simulink model "SSMM_sim_Torque_3DOF"  (R2020a)
settings: Solver=FixedStepAuto  StartTime=0.0  StopTime=120  FixedStep=0.001  MaxStep=1e-1  MinStep=1e-15  RelTol=.01  AbsTol=.01  EnableMultiTasking=on
InitFcn:
  | SSMM_sim_Torque_3DOF_Init
values from neighbouring files (symbols this model uses):
  CP_Num = CP_Base_Num + CP_Wheels_Num    [JACKAL_dynamic_model.m]
  D = D(:)    [ANFISFcn.m]    (also in JACKAL_dynamic_model.m = 1000)
  K = 1e6    (= 1000000)    [JACKAL_dynamic_model.m]
  model = floatbase(model)    [JACKAL_dynamic_model.m]
  Mu = .8    (= 0.8)    [JACKAL_dynamic_model.m]
  path = [      0         0 ... (first row only)    [JACKAL_dynamic_model.m]
  q_init = [0 0 0 0]'    [JACKAL_dynamic_model.m]
  qd_init = [0 0 0 0]'    [JACKAL_dynamic_model.m]
  R = .1    (= 0.1)    [JACKAL_dynamic_model.m]    (also in R.mat)
  speed = 1.5    [JACKAL_dynamic_model.m]
  width = basesize(2)    [JACKAL_dynamic_model.m]
  x_init = [1 0 0 0  0 0 zoff   0 0 0  2 0 0]'    [JACKAL_dynamic_model.m]
undefined symbols (not defined in the file or in its folder): DiscIntNeverNeededParam, Fpt, gcontact, gcPosVel
libraries: simulink x6, fuzblock x1
settings Model: Creator=Sergio  LastModifiedBy=sky32
settings SolverCC: MaxConsecutiveMinStep=5  AutoInsertRateTranBlk=on
settings DataIOCC: SaveFormat=Array  SignalLoggingSaveFormat=ModelDataLogs  ReturnWorkspaceOutputs=off
settings OptimizationCC: ExpressionDepthLimit=2147483647  LifeSpan=inf
settings DebuggingCC: UnderspecifiedInitializationDetection=Classic  MergeDetectMultiDrivingBlocksExec=none  SolverPrmCheckMsg=warning  MultiTaskDSMMsg=warning  MultiTaskCondExecSysMsg=none  StateNameClashWarn=warning  SFUnexpectedBacktrackingDiag=warning  SFNoUnconditionalDefaultTransitionDiag=warning  SFExecutionAtInitializationDiag=none  ArithmeticOperatorsInVariantConditions=warning
settings HardwareCC: ProdBitPerPointer=32  ProdBitPerSizeT=32  ProdBitPerPtrDiffT=32  ProdLargestAtomicFloat=None  ProdIntDivRoundTo=Undefined  ProdEndianess=Unspecified  ProdWordSize=32  ProdHWDeviceType=32-bit Generic
settings ModelReferenceCC: PropagateSignalLabelsOutOfModel=off
settings SFSimCC: SimUseLocalCustomCode=off  CustomCodeUndefinedFunction=UseInterfaceOnly
settings RTWCC: RTWUseLocalCustomCode=off
settings CodeAppCC: StateflowObjectComments=on
settings GRTTargetCC: TargetLangStandard=C89/C90 (ANSI)
settings ConfigComp: CovMetricSettings=dw  CovHtmlReporting=on  CovSaveCumulativeToWorkspaceVar=on  CovSaveSingleToWorkspaceVar=on  CovExternalEMLEnable=off

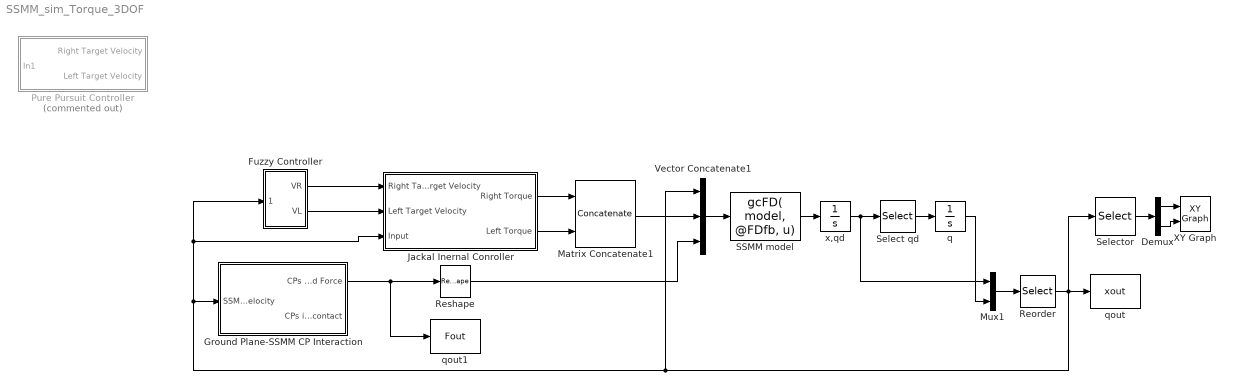
== system SSMM_sim_Torque_3DOF ==
  Demux : Demux  Outputs=2
  Fuzzy Controller : Subsystem
  Ground Plane-SSMM CP Interaction : Subsystem
  Jackal Inernal Conroller : Subsystem
  Matrix Concatenate1 : Concatenate  Mode=Multidimensional array
  Mux1 : Mux  Inputs=2
  Pure Pursuit Controller : Subsystem  Commented=on
  Reorder : Selector  InputPortWidth=21  IndexOptions=Index vector (dialog)  Indices=[1 2 3 4 5 6 7 8 9 10 11 12 13 18 19 20 21 14 15 16 17]  OutputSizes=1
  Reshape : Reshape  OutputDimensionality=Column vector (2-D)
  SSMM model : MATLABFcn  MATLABFcn=gcFD( model, @FDfb, u)  OutputDimensions=[17 1]  OutputSignalType=real  Output1D=off
  Select qd : Selector  InputPortWidth=17  IndexOptions=Index vector (dialog)  Indices=[14 15 16 17]  OutputSizes=1
  Selector : Selector  InputPortWidth=21  IndexOptions=Index vector (dialog)  Indices=[5 6]  OutputSizes=1
  Vector Concatenate1 : Concatenate  NumInputs=3
  XY Graph : simulink/Sinks/XY Graph  xmin=-10  xmax=20  ymin=-20  ymax=10  st=-1
  q : Integrator  InitialCondition=q_init
  qout : ToWorkspace  VariableName=xout  SampleTime=-1
  qout1 : ToWorkspace  VariableName=Fout  SampleTime=-1
  x,qd : Integrator  InitialCondition=[x_init;qd_init]
  wires:
  Vector Concatenate1/1 -> SSMM model/1
  SSMM model/1 -> x,qd/1
  Reshape/1 -> Vector Concatenate1/3
  x,qd/1 -> Select qd/1, Mux1/1
  Select qd/1 -> q/1
  Mux1/1 -> Reorder/1
  q/1 -> Mux1/2
  Ground Plane-SSMM CP Interaction/1(CPs Applied Force) -> qout1/1, Reshape/1
  Matrix Concatenate1/1 -> Vector Concatenate1/2
  Jackal Inernal Conroller/1(Right Torque) -> Matrix Concatenate1/1
  Jackal Inernal Conroller/2(Left Torque) -> Matrix Concatenate1/2
  Demux/2 -> XY Graph/2
  Selector/1 -> Demux/1
  Demux/1 -> XY Graph/1
  Reorder/1 -> Vector Concatenate1/1, Ground Plane-SSMM CP Interaction/1(SSMM Position and Velocity), Fuzzy Controller/1(theta,x,y), Jackal Inernal Conroller/3(Input), Selector/1, qout/1
  Fuzzy Controller/1(VR) -> Jackal Inernal Conroller/1(Right Target Velocity)
  Fuzzy Controller/2(VL) -> Jackal Inernal Conroller/2(Left Target Velocity)

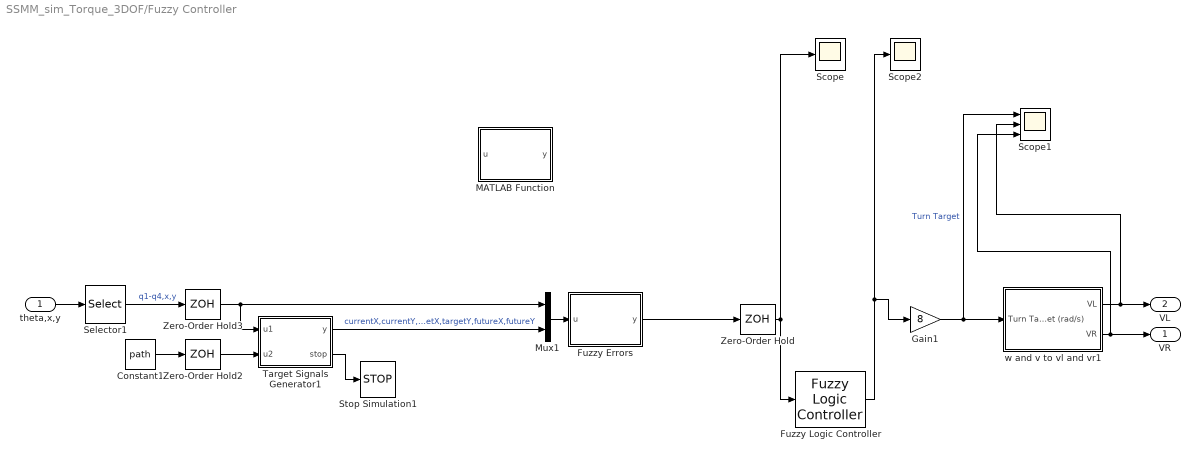
== system SSMM_sim_Torque_3DOF/Fuzzy Controller ==
  theta,x,y : Inport
  Constant1 : Constant  Value=path
  Fuzzy Errors : MATLAB Function  TreatAsAtomicUnit=on
  Fuzzy Logic Controller : fuzblock/Fuzzy Logic  Controller  FIS='fuzzycontrolthreeinputs6'  OutputSampleNumber=101  DataType=double  FuzzifiedInputs=off  RuleFiringStrengths=off  RuleOutputs=off  AggregatedOutputs=off  SimulateUsing=Interpreted execution  OutOfRangeInputValueMessage=warning  NoRuleFiredMessage=warning  EmptyOutputFuzzySetMessage=warning
  Gain1 : Gain  Gain=8
  MATLAB Function : MATLAB Function  TreatAsAtomicUnit=on
  Mux1 : Mux  Inputs=2
  Scope : Scope
  Scope1 : Scope  NumInputPorts=3
  Scope2 : Scope
  Selector1 : Selector  InputPortWidth=21  IndexOptions=Index vector (dialog)  Indices=[1 2 3 4 5 6]  OutputSizes=1
  Stop Simulation1 : Stop
  Target Signals Generator1 : MATLAB Function  TreatAsAtomicUnit=on
  Zero-Order Hold : ZeroOrderHold  SampleTime=.001
  Zero-Order Hold2 : ZeroOrderHold  SampleTime=.001
  Zero-Order Hold3 : ZeroOrderHold  SampleTime=.001
  w and v to vl and vr1 : Subsystem
  VR : Outport  VectorParamsAs1DForOutWhenUnconnected=off
  VL : Outport  Port=2  VectorParamsAs1DForOutWhenUnconnected=off
  wires:
  theta,x,y/1 -> Selector1/1
  Mux1/1 -> Fuzzy Errors/1(u)
  Fuzzy Logic Controller/1 -> Scope2/1, Gain1/1
  Zero-Order Hold3/1 -> Target Signals Generator1/1(u1), Mux1/1
  Selector1/1 -> Zero-Order Hold3/1  "q1-q4,x,y"
  Target Signals Generator1/1(y) -> Mux1/2  "currentX,currentY,targetX,targetY,futureX,futureY"
  Constant1/1 -> Zero-Order Hold2/1
  w and v to vl and vr1/2(VR) -> VR/1, Scope1/3
  Zero-Order Hold2/1 -> Target Signals Generator1/2(u2)
  Target Signals Generator1/2(stop) -> Stop Simulation1/1
  w and v to vl and vr1/1(VL) -> VL/1, Scope1/2
  Gain1/1 -> Scope1/1, w and v to vl and vr1/1(Turn Target (rad/s))  "Turn Target"
  Fuzzy Errors/1(y) -> Zero-Order Hold/1
  Zero-Order Hold/1 -> Fuzzy Logic Controller/1, Scope/1

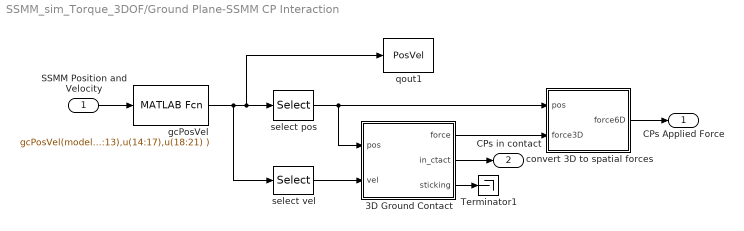
== system SSMM_sim_Torque_3DOF/Ground Plane-SSMM CP Interaction ==
  SSMM Position and Velocity : Inport
  3D Ground Contact : Subsystem  mask(3D Nonlinear Ground Contact with Friction){K=K, D=D, mu=Mu, np=CP_Num}
      mask prompts: K "Stiffness (K)"; D "Damping (D)"; mu "Coefficient of Friction (mu)"; np "Number of Contact Points"
      mask help:
      | Given two 3xnp arrays containing contact-point positions and
      | velocities, calculate the 3xnp array of ground-reaction forces
      | acting on those points. Also calculate 1xnp boolean vectors
      | in_ctact (true if normal force >0) and sticking (true if inside
      | or on boundary of friction cone).  Zero-crossing detection is
      | enabled at both make/break contact and stick/slip transitions.
  Terminator1 : Terminator
  convert 3D to spatial forces : Subsystem
  gcPosVel : MATLABFcn  MATLABFcn=gcPosVel(model, u(1:13),u(14:17),u(18:21) )  OutputDimensions=[6 CP_Num]  OutputSignalType=real  Output1D=off
  qout1 : ToWorkspace  VariableName=PosVel  SampleTime=-1
  select pos : Selector  NumberOfDimensions=2  InputPortWidth=3  IndexOptions=Index vector (dialog),Select all  Indices=[1 2 3],1  OutputSizes=1,1
  select vel : Selector  NumberOfDimensions=2  InputPortWidth=3  IndexOptions=Index vector (dialog),Select all  Indices=[4 5 6],1  OutputSizes=1,1
  CPs Applied Force : Outport  VectorParamsAs1DForOutWhenUnconnected=off
  CPs in contact : Outport  Port=2  VectorParamsAs1DForOutWhenUnconnected=off
  wires:
  gcPosVel/1 -> select vel/1, qout1/1, select pos/1
  select pos/1 -> convert 3D to spatial forces/1(pos), 3D Ground Contact/1(pos)
  convert 3D to spatial forces/1(force6D) -> CPs Applied Force/1
  select vel/1 -> 3D Ground Contact/2(vel)
  3D Ground Contact/3(sticking) -> Terminator1/1
  3D Ground Contact/2(in_ctact) -> CPs in contact/1
  SSMM Position and Velocity/1 -> gcPosVel/1
  3D Ground Contact/1(force) -> convert 3D to spatial forces/2(force3D)

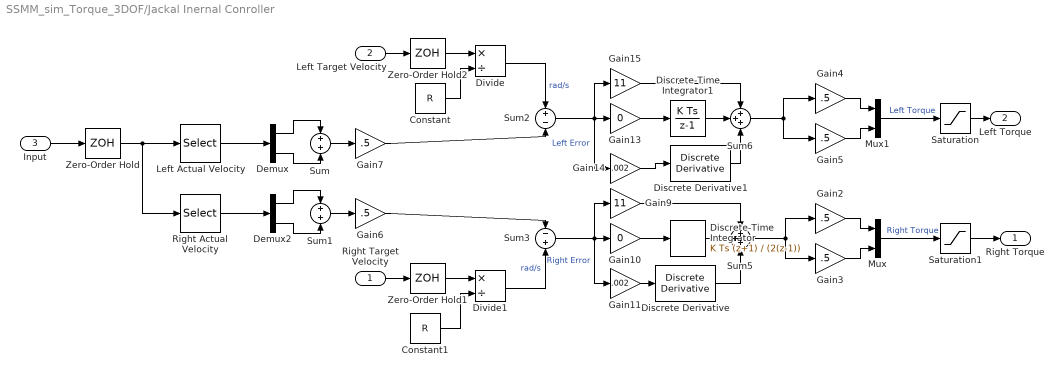
== system SSMM_sim_Torque_3DOF/Jackal Inernal Conroller ==
  Right Target Velocity : Inport
  Left Target Velocity : Inport  Port=2
  Input : Inport  Port=3
  Constant : Constant  Value=R
  Constant1 : Constant  Value=R
  Demux : Demux  Outputs=2
  Demux2 : Demux  Outputs=2
  Discrete Derivative : simulink/Discrete/Discrete Derivative  gainval=1  ICPrevScaledInput=0.0  OutMin=[]  OutMax=[]  OutDataType=fixdt(1, 16)  OutScaling=2^-10  DoSatur=off
  Discrete Derivative1 : simulink/Discrete/Discrete Derivative  gainval=1  ICPrevScaledInput=0.0  OutMin=[]  OutMax=[]  OutDataType=fixdt(1, 16)  OutScaling=2^-10  DoSatur=off
  Discrete-Time Integrator : DiscreteIntegrator  IntegratorMethod=Integration: Trapezoidal  SampleTime=-1  ICPrevOutput=DiscIntNeverNeededParam  ICPrevScaledInput=DiscIntNeverNeededParam
  Discrete-Time Integrator1 : DiscreteIntegrator  SampleTime=-1  ICPrevOutput=DiscIntNeverNeededParam  ICPrevScaledInput=DiscIntNeverNeededParam
  Divide : Product  Inputs=*/
  Divide1 : Product  Inputs=*/
  Gain10 : Gain  Gain=0
  Gain11 : Gain  Gain=.002
  Gain13 : Gain  Gain=0
  Gain14 : Gain  Gain=.002
  Gain15 : Gain  Gain=11
  Gain{2..7} (6 alike) : Gain  Gain=.5
  Gain9 : Gain  Gain=11
  Left Actual Velocity : Selector  InputPortWidth=21  IndexOptions=Index vector (dialog)  Indices=[20 21]  OutputSizes=1
  Mux : Mux  Inputs=2
  Mux1 : Mux  Inputs=2
  Right Actual Velocity : Selector  InputPortWidth=21  IndexOptions=Index vector (dialog)  Indices=[18 19]  OutputSizes=1
  Saturation : Saturate  UpperLimit=1000  LowerLimit=-1000
  Saturation1 : Saturate  UpperLimit=1000  LowerLimit=-1000
  Sum : Sum  Inputs=2
  Sum1 : Sum  Inputs=2
  Sum2 : Sum  Inputs=+-
  Sum3 : Sum  Inputs=-+
  Sum5 : Sum  Inputs=+++
  Sum6 : Sum  Inputs=+++
  Zero-Order Hold : ZeroOrderHold  SampleTime=.001
  Zero-Order Hold1 : ZeroOrderHold  SampleTime=.001
  Zero-Order Hold2 : ZeroOrderHold  SampleTime=.001
  Right Torque : Outport  VectorParamsAs1DForOutWhenUnconnected=off
  Left Torque : Outport  Port=2  VectorParamsAs1DForOutWhenUnconnected=off
  wires:
  Gain3/1 -> Mux/2
  Input/1 -> Zero-Order Hold/1
  Left Actual Velocity/1 -> Demux/1
  Demux/1 -> Sum/1
  Demux/2 -> Sum/2
  Demux2/1 -> Sum1/1
  Demux2/2 -> Sum1/2
  Right Actual Velocity/1 -> Demux2/1
  Sum1/1 -> Gain6/1
  Sum/1 -> Gain7/1
  Gain6/1 -> Sum3/1
  Sum3/1 -> Gain9/1, Gain11/1, Gain10/1  "Right Error"
  Gain9/1 -> Sum5/1
  Gain10/1 -> Discrete-Time Integrator/1
  Gain4/1 -> Mux1/1
  Gain5/1 -> Mux1/2
  Left Target Velocity/1 -> Zero-Order Hold2/1
  Constant/1 -> Divide/2
  Divide/1 -> Sum2/1  "rad/s"
  Constant1/1 -> Divide1/2
  Divide1/1 -> Sum3/2  "rad/s"
  Gain7/1 -> Sum2/2
  Gain2/1 -> Mux/1
  Mux1/1 -> Saturation/1  "Left Torque"
  Mux/1 -> Saturation1/1  "Right Torque"
  Sum5/1 -> Gain3/1, Gain2/1
  Zero-Order Hold/1 -> Right Actual Velocity/1, Left Actual Velocity/1
  Right Target Velocity/1 -> Zero-Order Hold1/1
  Zero-Order Hold1/1 -> Divide1/1
  Zero-Order Hold2/1 -> Divide/1
  Gain11/1 -> Discrete Derivative/1
  Discrete Derivative/1 -> Sum5/3
  Discrete-Time Integrator/1 -> Sum5/2
  Gain14/1 -> Discrete Derivative1/1
  Gain13/1 -> Discrete-Time Integrator1/1
  Sum2/1 -> Gain15/1, Gain14/1, Gain13/1  "Left Error"
  Discrete Derivative1/1 -> Sum6/3
  Sum6/1 -> Gain5/1, Gain4/1
  Gain15/1 -> Sum6/1
  Discrete-Time Integrator1/1 -> Sum6/2
  Saturation/1 -> Left Torque/1
  Saturation1/1 -> Right Torque/1

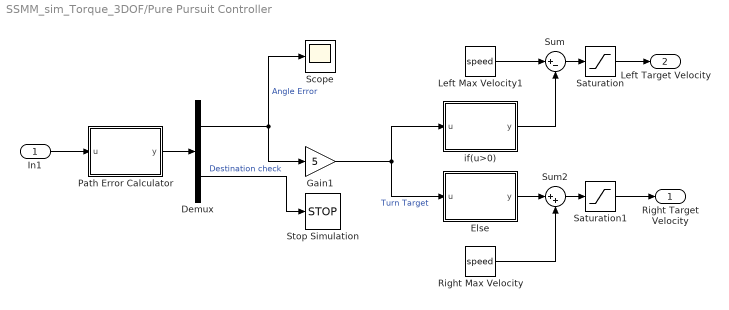
== system SSMM_sim_Torque_3DOF/Pure Pursuit Controller ==
  In1 : Inport
  Demux : Demux  Outputs=2
  Else : MATLAB Function  TreatAsAtomicUnit=on
  Gain1 : Gain  Gain=5
  Left Max Velocity1 : Constant  Value=speed
  Path Error Calculator : MATLAB Function  TreatAsAtomicUnit=on
  Right Max Velocity : Constant  Value=speed
  Saturation : Saturate  UpperLimit=speed  LowerLimit=-speed
  Saturation1 : Saturate  UpperLimit=speed  LowerLimit=-speed
  Scope : Scope
  Stop Simulation : Stop
  Sum : Sum  Inputs=|+-
  Sum2 : Sum  Inputs=|++
  if(u>0) : MATLAB Function  TreatAsAtomicUnit=on
  Right Target Velocity : Outport  VectorParamsAs1DForOutWhenUnconnected=off
  Left Target Velocity : Outport  Port=2  VectorParamsAs1DForOutWhenUnconnected=off
  wires:
  Path Error Calculator/1(y) -> Demux/1
  In1/1 -> Path Error Calculator/1(u)
  Gain1/1 -> if(u>0)/1(u), Else/1(u)  "Turn Target"
  Left Max Velocity1/1 -> Sum/1
  Right Max Velocity/1 -> Sum2/2
  if(u>0)/1(y) -> Sum/2
  Sum/1 -> Saturation/1
  Saturation/1 -> Left Target Velocity/1
  Sum2/1 -> Saturation1/1
  Saturation1/1 -> Right Target Velocity/1
  Demux/2 -> Stop Simulation/1  "Destination check"
  Demux/1 -> Scope/1, Gain1/1  "Angle Error"
  Else/1(y) -> Sum2/1

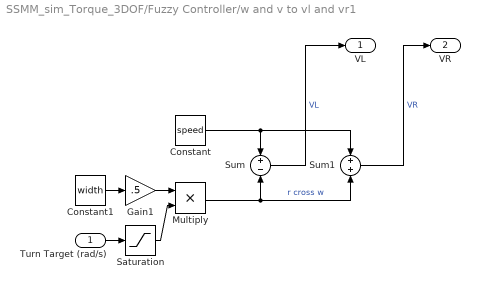
== system SSMM_sim_Torque_3DOF/Fuzzy Controller/w and v to vl and vr1 ==
  Turn Target (rad/s) : Inport
  Constant : Constant  Value=speed
  Constant1 : Constant  Value=width
  Gain1 : Gain  Gain=.5
  Multiply : Product  Inputs=**
  Saturation : Saturate  UpperLimit=4  LowerLimit=-4
  Sum : Sum  Inputs=+|-
  Sum1 : Sum  Inputs=+|+
  VL : Outport  VectorParamsAs1DForOutWhenUnconnected=off
  VR : Outport  Port=2  VectorParamsAs1DForOutWhenUnconnected=off
  wires:
  Multiply/1 -> Sum/2, Sum1/2  "r cross w"
  Sum1/1 -> VR/1  "VR"
  Sum/1 -> VL/1  "VL"
  Constant1/1 -> Gain1/1
  Gain1/1 -> Multiply/1
  Constant/1 -> Sum1/1, Sum/1
  Turn Target (rad/s)/1 -> Saturation/1
  Saturation/1 -> Multiply/2

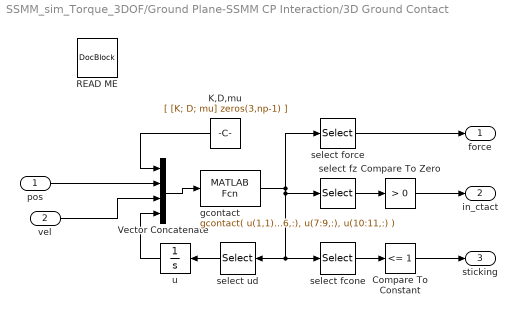
== system SSMM_sim_Torque_3DOF/Ground Plane-SSMM CP Interaction/3D Ground Contact ==
  pos : Inport
  vel : Inport  Port=2
  Compare To Constant : simulink/Logic and Bit Operations/Compare To Constant  relop=<=  const=1  OutDataTypeStr=boolean
  Compare To Zero : simulink/Logic and Bit Operations/Compare To Zero  relop=>  OutDataTypeStr=boolean
  K,D,mu : Constant  Value=[ [K; D; mu] zeros(3,np-1) ]  VectorParams1D=off
  READ ME : simulink/Model-Wide Utilities/DocBlock  DocumentType=Text
      content=|
      | The constant block supplies the parameters K, D and mu to the function
      | gcontact.  This is necessary because K, D and mu are defined in the
      | workspace of this particular masked subsystem, but the executable
      | expression in the "MATLAB Function" block does not have access to this
      | workspace, so the symbols K, D and mu cannot appear directly in the
      | executable expression.
      |
      | The ">0" block and the "<=1" block both have zero-crossing enabled.  The
      | former detects transitions between contact and non-contact, whereas the
      | latter detects transitions between sticking (due to friction) and
      | slipping.  A point can be sticking only if it is also in contact.  A
      | zero-crossing event occurs whenever any one point makes a transition.
      |
      | The state variable, u, is a 2x(np) matrix containing the horizontal
      | component of the local ground deformation for each point.  This quantity
      | is used to calculate the tangential (i.e., frictional) component of the
      | ground reaction force.
      |
      | When a point loses contact, its associated state variable, u(:,i), decays
      | to zero with a time constant of D/K.  If this ratio is small then the
      | corresponding differential equation is fast, and it is necessary to use
      | small integration time steps.  For example, if K=1e6 and D=2000 then
      | D/K=0.002 and u(:,i) decays in proportion to exp(-500t).  Increasing K
      | makes the surface stiffer, and decreasing D/K makes it bouncier, but the
      | latter also makes the post-contact recovery faster.  The degree of
      | bounciness depends on the mass of the impacting body: a heavier body will
      | bounce more.
      |
      | To adapt this subsystem to work in 2D, the only things that change are the
      | row dimensions of various matrices.  You will have to alter the row
      | selections in the executable expression in the "MATLAB Function" block,
      | and also the dimensions of its output matrix, and you will have to change
      | the row selections in the various "select" blocks.
      |
      | For more information, see "The Simulink Ground Contact Model" in the
      | spatial_v2 documentation directory.
  Vector Concatenate : Concatenate  NumInputs=4  Mode=Multidimensional array
  gcontact : MATLABFcn  MATLABFcn=gcontact( u(1,1), u(2,1), u(3,1), u(4:6,:), u(7:9,:), u(10:11,:) )  OutputDimensions=[6 np]  OutputSignalType=real  Output1D=off
  select fcone : Selector  NumberOfDimensions=2  InputPortWidth=3  IndexOptions=Index vector (dialog),Select all  Indices=[6],1  OutputSizes=1,1
  select force : Selector  NumberOfDimensions=2  InputPortWidth=3  IndexOptions=Index vector (dialog),Select all  Indices=[1 2 3],1  OutputSizes=1,1
  select fz : Selector  NumberOfDimensions=2  InputPortWidth=3  IndexOptions=Index vector (dialog),Select all  Indices=[3],1  OutputSizes=1,1
  select ud : Selector  NumberOfDimensions=2  InputPortWidth=3  IndexOptions=Index vector (dialog),Select all  Indices=[4 5],1  OutputSizes=1,1
  u : Integrator
  force : Outport  VectorParamsAs1DForOutWhenUnconnected=off
  in_ctact : Outport  Port=2  VectorParamsAs1DForOutWhenUnconnected=off
  sticking : Outport  Port=3  VectorParamsAs1DForOutWhenUnconnected=off
  wires:
  Vector Concatenate/1 -> gcontact/1
  select ud/1 -> u/1
  gcontact/1 -> select fz/1, select ud/1, select fcone/1, select force/1
  select fz/1 -> Compare To Zero/1
  select fcone/1 -> Compare To Constant/1
  Compare To Constant/1 -> sticking/1
  u/1 -> Vector Concatenate/4
  pos/1 -> Vector Concatenate/2
  K,D,mu/1 -> Vector Concatenate/1
  vel/1 -> Vector Concatenate/3
  Compare To Zero/1 -> in_ctact/1
  select force/1 -> force/1

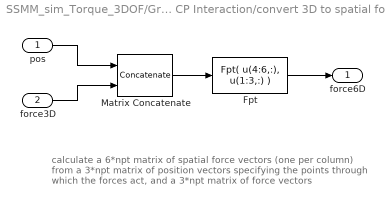
== system SSMM_sim_Torque_3DOF/Ground Plane-SSMM CP Interaction/convert 3D to spatial forces ==
  note: calculate a 6*npt matrix of spatial force vectors (one per column)
      | from a 3*npt matrix of position vectors specifying the points
      | through which the forces act, and a 3*npt matrix of force vectors
  pos : Inport
  force3D : Inport  Port=2
  Fpt : MATLABFcn  MATLABFcn=Fpt( u(4:6,:), u(1:3,:) )  OutputSignalType=real  Output1D=off
  Matrix Concatenate : Concatenate  Mode=Multidimensional array
  force6D : Outport  VectorParamsAs1DForOutWhenUnconnected=off
  wires:
  force3D/1 -> Matrix Concatenate/2
  pos/1 -> Matrix Concatenate/1
  Matrix Concatenate/1 -> Fpt/1
  Fpt/1 -> force6D/1

== matlab function SSMM_sim_Torque_3DOF/Pure Pursuit Controller/Path Error Calculator ==
  data: u input; y output
%the goal of this script is to check where the robot needs to go (via
%looking at path stepoints) and if the robot needs to travel towards a
%setpoint, it calculates the difference between the robot's actual heading
%and what its desired heading should be to reach that point while traveling
%in a straight line.

function y = fcn(u)
coder.extrinsic('evalin', 'assignin');
pathcount = 0; pathlength=0; % Needed in order to set variable class correctly

pathcount = evalin('base','pathcount'); % Read pathcount from workspace             
pathlength = evalin('base','pathlength'); % Read pathlength from workspace   

path=zeros(pathlength,2);
path = evalin('base','path'); % Read path from workspace

pathflag=0; %flag to stop sim when all points are reached
[len,~]=size(path);
path=[path; 500 500];

pos=[u(5) u(6)]; % [x,y]
q=[u(1) u(2) u(3) u(4)]; % orientation quaternion

target=path(pathcount+1,:); %target point is the next point in the path
distErr=sqrt((target(1)-pos(1))^2+(target(2)-pos(2))^2);

if(distErr<.35)
    pathcount=pathcount+1;
    target=path(pathcount+1,:);
    assignin('base','pathcount',pathcount); % Assign new pathcount back to workspace
end

targetAngle=atan2(target(2)-pos(2),target(1)-pos(1)); % Angle between current robot position and the target
currentAngle=atan2(2*(q(1)*q(4)+q(2)*q(3)),1-2*(q(3)^2+q(4)^2));% Angle robot is currently facing
angErr=targetAngle-currentAngle;
    
if(angErr>pi()) %keep error between -pi and pi
    angErr=angErr-2*pi();
end

if(angErr<(-1*pi()))
    angErr=angErr+2*pi();
end

if(pathcount>=len) %if all of the target points have been reached
    pathflag=1;
end

y=[angErr pathflag];

== matlab function SSMM_sim_Torque_3DOF/Fuzzy Controller/MATLAB Function ==
  data: u input; y output
function y = fcn(u)
coder.extrinsic('evalin','assignin','py.hi1.abc','py.load_agent.ddpg')
anfis = evalin('base', 'anfis');

action = 0;
%mod
persistent flag;
if isempty(flag)
    flag = false;
    anfis = py.load_agent.ddpg();
    action = py.hi1.abc(u(1),u(2),u(3),anfis)
    
end

if flag == true 
    action = py.hi1.abc(u(1),u(2),u(3),anfis);
end
assignin('base', 'anfis', anfis);
flag = true;

y = action;

== matlab function SSMM_sim_Torque_3DOF/Pure Pursuit Controller/if(u>0) ==
  data: u input; y output
function y = fcn(u)
if(u>0)
    y = u;
else
    y=0;
end

== matlab function SSMM_sim_Torque_3DOF/Pure Pursuit Controller/Else ==
  data: u input; y output
function y = fcn(u)
if(u<=0)
    y=u;
else
    y=0;
end

== matlab function SSMM_sim_Torque_3DOF/Fuzzy Controller/Fuzzy Errors ==
  settings: updateMethod=DISCRETE
  data: u input; y output
function y  = fcn(u)

%jackal dyanamic model
pos=[u(5) u(6)]; % [x,y]
q=[u(1) u(2) u(3) u(4)]; % orientation quaternion
currentAngle=atan2(2*(q(1)*q(4)+q(2)*q(3)),1-2*(q(3)^2+q(4)^2));% Angle robot is currently facing

currentPoint=[u(7) u(8)];
target=[u(9) u(10)];
future=[u(11) u(12)];

A = [(currentPoint(2)-target(2)), target(1)-currentPoint(1); target(1)-currentPoint(1), target(2)-currentPoint(2)];
b = [ target(1)*currentPoint(2)-currentPoint(1)*target(2); pos(1)*(target(1)-currentPoint(1)) + pos(2)*(target(2)-currentPoint(2))];
proj = (A\b)'; %projected point on the line between  .

d = ( pos(1)-currentPoint(1) )*(target(2)-currentPoint(2)) - (pos(2)-currentPoint(2))*(target(1)-currentPoint(1));

if ( d >0)
    side = 1;
elseif ( d < 0)
    side = -1;
else
    side = 0;
end

distanceLine=norm(pos-proj)*side;
distanceTarget=sqrt((target(1)-pos(1))^2+(target(2)-pos(2))^2);

%wrap to +/-pi
if((currentAngle < -pi) || (pi < currentAngle))
    currentAngle = mod(currentAngle+pi, 2*pi)-pi;
end

farTarget=[.9*proj(1)+.1*target(1) .9*proj(2)+.1*target(2)];

th1 = atan2(farTarget(2)-pos(2), farTarget(1)-pos(1));
th2 = atan2(target(2)-currentPoint(2), target(1)-currentPoint(1));
th3 = atan2(future(2)-target(2), future(1)-target(1)); 

ThetaFar=th1-currentAngle;
ThetaNear=th2-currentAngle;
ThetaLookahead=th3-currentAngle;

%wrap to +/-pi
if((ThetaFar < -pi) || (pi < ThetaFar))
    ThetaFar = mod(ThetaFar+pi, 2*pi)-pi;
end

%wrap to +/-pi
if((ThetaNear < -pi) || (pi < ThetaNear))
    ThetaNear = mod(ThetaNear+pi, 2*pi)-pi;
end

%wrap to +/-pi
if((ThetaLookahead < -pi) || (pi < ThetaLookahead))
    ThetaLookahead = mod(ThetaLookahead+pi, 2*pi)-pi;
end

%y = [distanceLine;ThetaFar;ThetaNear;ThetaLookahead;distanceTarget]; 
y = [distanceLine;ThetaFar;ThetaNear];

== matlab function SSMM_sim_Torque_3DOF/Fuzzy Controller/Target Signals Generator1 ==
  data: u1 input; y output; u2 input; stop output
function [y,stop] = fcn(u1,u2)

persistent pathcount;
persistent pathlength;
persistent path; %error in code, initially used path but this is already a matlab function
persistent pathPre;

if isempty(pathcount)
   pathcount=1;     
   pathPre=u2;
   [pathlength,~]=size(pathPre);  
   path=[pathPre; pathPre(pathlength,1)+100 pathPre(pathlength,2)+100]; %sim takes multiple iterations to stop after reaching final point, so this prevents it from breaking
end

pos=[u1(5) u1(6)]; % [x,y] 
currentPoint=path(pathcount,:);
target=path(pathcount+1,:);

A = [(currentPoint(2)-target(2)), target(1)-currentPoint(1); target(1)-currentPoint(1), target(2)-currentPoint(2)];
b = [ target(1)*currentPoint(2)-currentPoint(1)*target(2); pos(1)*(target(1)-currentPoint(1)) + pos(2)*(target(2)-currentPoint(2))];
proj = (A\b)'; %projected point on the line between  .
projLen=dot(proj-currentPoint,target-currentPoint)/norm(target-currentPoint)^2; %the distance along the projected line, where 0 is the start point and 1 is the end point

if ((projLen>1))
    pathcount=pathcount+1;
end

%check if at destination and terminate sim if there
pathflag=0;
if (pathcount==pathlength)
    
    pathflag=1;
end

if ((pathcount==(pathlength-1))||(pathcount==(pathlength)))
    a=path(pathcount,:);
    b=path(pathcount+1,:);
    post=path(pathcount+1,:);
else
    a=path(pathcount,:);
    b=path(pathcount+1,:);
    post=path(pathcount+2,:);
end

y = [a(1);a(2);b(1);b(2);post(1);post(2)];
stop=pathflag;
